simulink model "tubulaoNL"  (R2018b)
settings: Solver=VariableStepAuto  StartTime=0.0  StopTime=30  RelTol=1e-3
undefined symbols (not defined in the file): l, magnitude, R
settings Model: Creator=Aniel  LastModifiedBy=Aniel

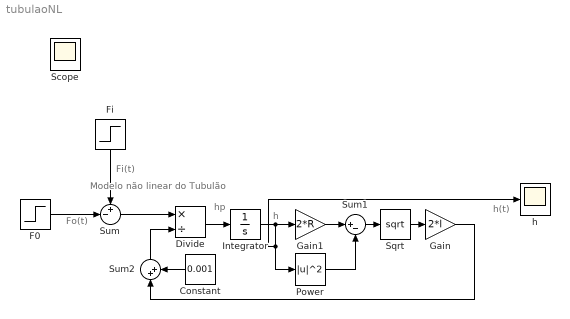
== system tubulaoNL ==
  note: h(t)
  note: Fo(t)
  note: Fi(t)
  note: Modelo não linear do Tubulão
  note: hp
  note: h
  Constant : Constant  Value=0.001
  Divide : Product  Inputs=*/
  F0 : Step  Time=20  SampleTime=0
  Fi : Step  SampleTime=0
  Gain : Gain  Gain=2*l
  Gain1 : Gain  Gain=2*R
  Integrator : Integrator
  Power : Math  Operator=magnitude^2  SaturateOnIntegerOverflow=on
  Sqrt : Sqrt  SaturateOnIntegerOverflow=on
  Sum : Sum  Inputs=+-|
  Sum1 : Sum  Inputs=|+-
  Sum2 : Sum  Inputs=|++
  h : Scope
  Scope : Scope
  wires:
  F0/1 -> Sum/2
  Fi/1 -> Sum/1
  Integrator/1 -> h/1, Power/1, Gain1/1
  Gain1/1 -> Sum1/1
  Power/1 -> Sum1/2
  Sum1/1 -> Sqrt/1
  Sqrt/1 -> Gain/1
  Sum/1 -> Divide/1
  Divide/1 -> Integrator/1
  Sum2/1 -> Divide/2
  Gain/1 -> Sum2/1
  Constant/1 -> Sum2/2
